simulink model "USART_Rcv_SoftInterrupt"  (R2013b)
settings: Solver=FixedStepDiscrete  StartTime=0.0  StopTime=10.0  FixedStep=0.5  RelTol=1e-3
undefined symbols (not defined in the file): PC10, PC11, uart4, usart3
libraries: USART_Lib x3, IT_Lib x1
settings Model: Creator=reynaudp  LastModifiedBy=reynaudp
settings SolverCC: AutoInsertRateTranBlk=on
settings OptimizationCC: ExpressionDepthLimit=2147483647  OptimizeModelRefInitCode=on  LifeSpan=1
settings DebuggingCC: StateNameClashWarn=warning
settings HardwareCC: ProdLargestAtomicInteger=Integer  ProdLargestAtomicFloat=Float  ProdIntDivRoundTo=Zero  ProdEndianess=LittleEndian  ProdHWDeviceType=STMicroelectronics->STM32F4xx 32-bit Cortex-M4
settings RTWCC: SystemTargetFile=stm32F4xx.tlc  TemplateMakefile=stm32F4xx.tmf  Description=stm32F4xx (Embedded Target)  GenerateReport=on  ProcessScript=stm32F4xx_make_rtw_hook  IncludeHyperlinkInReport=on  LaunchReport=on
settings CodeAppCC: IgnoreCustomStorageClasses=off  MaxIdLength=64  CustomSymbolStrType=$N$R$M  InternalIdentifier=Classic
settings STFCustomTargetCC: ParMdlRefBuildCompliant=on  IncludeMdlTerminateFcn=off  CombineOutputUpdateFcns=on  ERTCustomFileBanners=on  SupportContinuousTime=off  SupportNonInlinedSFcns=off  SupportVariableSizeSignals=on  MATLABClassNameForMDSCustomization=Simulink.SoftwareTarget.ERTCustomization  GRTInterface=off  SystemTargetFile=stm32F4xx.tlc
settings ERTTargetCC: CodeReplacementLibrary=ANSI_C  CompOptLevelCompliant=off  ConcurrentExecutionCompliant=off  IncludeMdlTerminateFcn=off  ERTFirstTimeCompliant=off  SupportVariableSizeSignals=on  ModelStepFunctionPrototypeControlCompliant=off  CPPClassGenCompliant=off  InlinedParameterPlacement=NonHierarchical  ERTSrcFileBannerTemplate=sourceFileTemplate.cgt  ERTHdrFileBannerTemplate=sourceFileTemplate.cgt  ERTDataSrcFileTemplate=sourceFileTemplate.cgt  ERTDataHdrFileTemplate=sourceFileTemplate.cgt  ERTCustomFileTemplate=customRoutineProcess.tlc

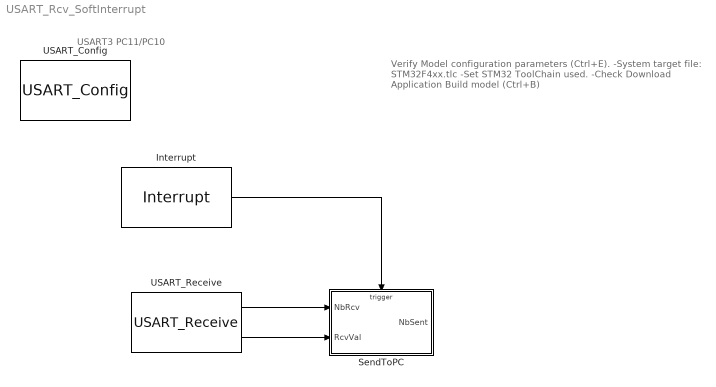
== system USART_Rcv_SoftInterrupt ==
  note: USART3 PC11/PC10
  note: Verify Model configuration parameters (Ctrl+E).
      | 	-System target file: STM32F4xx.tlc
      | 	-Set STM32 ToolChain used.
      | 	-Check Download Application
      | Build model (Ctrl+B)
  Interrupt : IT_Lib/Interrupt  Peripheral_name=EXTint  Peripheral_IRQid=11  Enable_sim=off  ADC1_en=on  ADC2_en=off  ADC3_en=off  ADC_EOC=off  ADC_JEOC=off  ADC_AWD=on  ADC_OVR=off  EXTI_port=GPIOA  EXTI_line=0  EXTI_trig=Rising  Def_handler=on  Cust_handler=EXTI0_IRQHandler  Group_prio=NVIC_PriorityGroup_0  Pre0_prio=0  Sub0_prio=0  Pre1_prio=0  Sub1_prio=0  Pre2_prio=0  Sub2_prio=0  Pre3_prio=0  Sub3_prio=0  Pre4_prio=0  Sub4_prio=0  Time_base=0.1
  SendToPC : Subsystem  TreatAsAtomicUnit=on
  USART_Config : USART_Lib/USART_Config  USART_CONFIG=USART3  USART_CONFIG_PIN=PC11/PC10 : (usart3 / uart4)  USART_SPEED=115200  USART_DATA=USART_WordLength_8b  USART_PARITY=USART_Parity_No  USART_STOP=USART_StopBits_1  USART_FLOW=off  USART_DEFAULT=off  It_rcv=on  It_send=on  Def_handler=on  Cust_handler=USART3_IRQHandler
  USART_Receive : USART_Lib/USART_Receive  USART_name=USART3  Buff_size=512  NbData_Size=20  Soft_it=on  Soft_num=0
  wires:
  Interrupt/1 -> SendToPC/Trigger
  USART_Receive/1 -> SendToPC/1(NbRcv)
  USART_Receive/2 -> SendToPC/2(RcvVal)

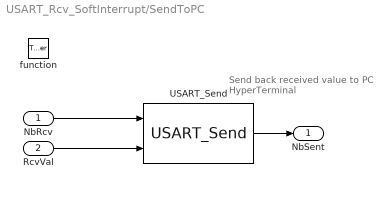
== system USART_Rcv_SoftInterrupt/SendToPC ==
  note: Send back received value to PC
      | HyperTerminal
  NbRcv : Inport  OutDataTypeStr=uint16
  RcvVal : Inport  Port=2
  function : TriggerPort  TriggerType=function-call
  USART_Send : USART_Lib/USART_Send  USART_name=USART3  USART_buff=20
  NbSent : Outport  OutDataTypeStr=uint16
  wires:
  NbRcv/1 -> USART_Send/1
  RcvVal/1 -> USART_Send/2
  USART_Send/1 -> NbSent/1
